simulink model "system_identification_project"  (R2020a)
settings: Solver=FixedStepAuto  StartTime=0.0  StopTime=600  FixedStep=0.01  RelTol=1e-3
libraries: cstblocks x1, simulink x1
settings Model: Creator=alejandropuerta  LastModifiedBy=elkin

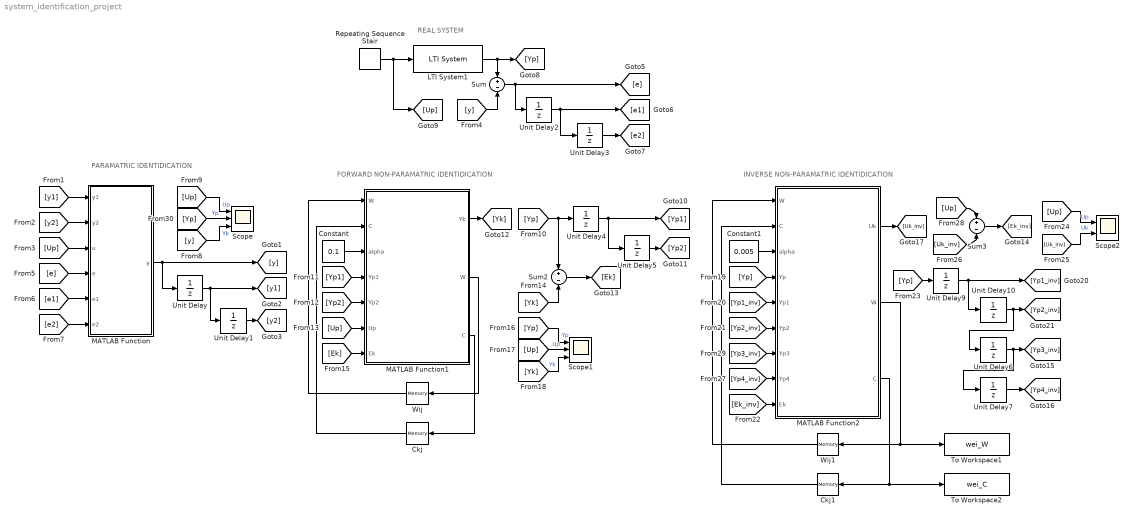
== system system_identification_project ==
  note: FORWARD NON-PARAMATRIC IDENTIDICATION
  note: PARAMATRIC IDENTIDICATION
  note: REAL SYSTEM
  note: INVERSE NON-PARAMATRIC IDENTIDICATION
  Ckj : Memory  InitialCondition=randn(1,10)
  Ckj1 : Memory  InitialCondition=randn(1,20)
  Constant : Constant  Value=0.1
  Constant1 : Constant  Value=0.005
  LTI System1 : cstblocks/LTI System  sys=servomotor  IC=[]
  MATLAB Function : MATLAB Function  TreatAsAtomicUnit=on
  MATLAB Function1 : MATLAB Function  TreatAsAtomicUnit=on
  MATLAB Function2 : MATLAB Function  TreatAsAtomicUnit=on
  Repeating Sequence Stair : simulink/Sources/Repeating Sequence Stair  OutValues=[0 0.2 0 0.4 0.8 0.4 1].'  tsamp=50  OutMin=[]  OutMax=[]  OutDataTypeStr=double  OutputDataTypeScalingMode=double  OutDataType=fixdt(0,8)  ConRadixGroup=Best Precision: Vector-wise  OutScaling=2^-12
  Scope : Scope  NumInputPorts=3
  Scope1 : Scope  NumInputPorts=3
  Scope2 : Scope  NumInputPorts=2
  Sum : Sum  Inputs=+-
  Sum2 : Sum  Inputs=+-
  Sum3 : Sum  Inputs=+-
  To Workspace1 : ToWorkspace  VariableName=wei_W  SampleTime=600
  To Workspace2 : ToWorkspace  VariableName=wei_C  SampleTime=600
  Unit Delay{,1..7,9..10} (10 alike) : UnitDelay  SampleTime=-1  HasFrameUpgradeWarning=on
  Wij : Memory  InitialCondition=randn(10,3)
  Wij1 : Memory  InitialCondition=randn(20,5)
  wires:
  LTI System1/1 -> Sum/1, [Yp]
  Repeating Sequence Stair/1 -> [Up], LTI System1/1
  MATLAB Function/1(y) -> [y], Unit Delay/1
  Unit Delay/1 -> [y1], Unit Delay1/1
  Unit Delay1/1 -> [y2]
  [y1] -> MATLAB Function/1(y1)
  [y2] -> MATLAB Function/2(y2)
  [Up] -> MATLAB Function/3(u)
  [y] -> Sum/2
  Sum/1 -> Unit Delay2/1, [e]
  Unit Delay2/1 -> Unit Delay3/1, [e1]
  Unit Delay3/1 -> [e2]
  [e] -> MATLAB Function/4(e)
  [e1] -> MATLAB Function/5(e1)
  [e2] -> MATLAB Function/6(e2)
  [y] -> Scope/3  "Yk"
  Constant/1 -> MATLAB Function1/3(alpha)
  [Yp] -> Unit Delay4/1, Sum2/1
  Unit Delay4/1 -> [Yp1], Unit Delay5/1
  Unit Delay5/1 -> [Yp2]
  [Yp1] -> MATLAB Function1/4(Yp1)
  [Yp2] -> MATLAB Function1/5(Yp2)
  [Up] -> MATLAB Function1/6(Up)
  MATLAB Function1/1(Yk) -> [Yk]
  [Yk] -> Sum2/2
  Sum2/1 -> [Ek]
  [Ek] -> MATLAB Function1/7(Ek)
  MATLAB Function1/2(W) -> Wij/1
  Wij/1 -> MATLAB Function1/1("W ")
  MATLAB Function1/3(C) -> Ckj/1
  Ckj/1 -> MATLAB Function1/2("C ")
  [Yp] -> Scope1/1  "Yp"
  [Up] -> Scope1/2  "Up"
  [Yk] -> Scope1/3  "Yk"
  Constant1/1 -> MATLAB Function2/3(alpha)
  MATLAB Function2/3(C) -> To Workspace2/1, Ckj1/1
  MATLAB Function2/2(W) -> Wij1/1, To Workspace1/1
  MATLAB Function2/1(Uk) -> [Uk_inv]
  Sum3/1 -> [Ek_inv]
  [Uk_inv] -> Sum3/2
  [Up] -> Sum3/1
  [Uk_inv] -> Scope2/2  "Uk"
  [Up] -> Scope2/1  "Up"
  Unit Delay9/1 -> [Yp1_inv], Unit Delay10/1
  [Yp] -> Unit Delay9/1
  Unit Delay10/1 -> Unit Delay6/1, [Yp2_inv]
  [Ek_inv] -> MATLAB Function2/9(Ek)
  [Yp2_inv] -> MATLAB Function2/6(Yp2)
  [Yp1_inv] -> MATLAB Function2/5(Yp1)
  [Yp] -> MATLAB Function2/4(Yp)
  [Yp4_inv] -> MATLAB Function2/8(Yp4)
  [Yp3_inv] -> MATLAB Function2/7(Yp3)
  Wij1/1 -> MATLAB Function2/1("W ")
  Ckj1/1 -> MATLAB Function2/2("C ")
  Unit Delay6/1 -> Unit Delay7/1, [Yp3_inv]
  Unit Delay7/1 -> [Yp4_inv]
  [Up] -> Scope/1  "Up"
  [Yp] -> Scope/2  "Yp"

== matlab function system_identification_project/MATLAB Function1 ==
  data: W input; Yk output; C input; alpha input; Yp1 input; Yp2 input; Up input; Ek input; W output; C output
function [Yk, W, C] = fcn(W, C, alpha, Yp1, Yp2, Up, Ek)
    % Define input vector
    X = [Yp1 Yp2 Up];
    
    % Calculate Aj in the hidden layer
    Aj = W*X';
    
    % Activation function of the hidden layer
    H = tanh(Aj);
    
    % Calculate Ak in the output layer
    Ak = C'*H;
    
    % Activation function of the output layer
    Yk = Ak;
    
    % Update C matrix
    C = C + alpha*Ek*H;
    
    % Update W matrix
    Hd = sech(Aj).^2;
    W = W + alpha*Ek*(C.*Hd)*X;

== matlab function system_identification_project/MATLAB Function ==
  data: y1 input; y2 input; u input; y output; e input; e1 input; e2 input
function y = fcn(y1,y2,u,e,e1,e2)

a1 = 1.9968;
a2 = -0.9968;
a3 = 1.3544e-05;
a4 = -1.7281;
a5 = 0.7410;

y = a1*y1 + a2*y2 + a3*u + e + a4*e1 + a5*e2;

== matlab function system_identification_project/MATLAB Function2 ==
  data: W input; Uk output; C input; alpha input; Yp input; Yp1 input; Yp2 input; Yp3 input; Yp4 input; Ek input; W output; C output
function [Uk, W, C] = fcn(W, C, alpha, Yp, Yp1, Yp2, Yp3, Yp4, Ek)
    % Define input vector
    X = [Yp Yp1 Yp2 Yp3 Yp4];
    
    % Calculate Aj in the hidden layer
    Aj = W*X';
    
    % Activation function of the hidden layer
    H = tanh(Aj);
    
    % Calculate Ak in the output layer
    Ak = C'*H;
    
    % Activation function of the output layer
    Uk = Ak;
    
    % Update C matrix
    C = C + alpha*Ek*H;
    
    % Update W matrix
    Hd = sech(Aj).^2;
    W = W + alpha*Ek*(C.*Hd)*X;
